simulink model "vehicle_spped_control_through_gear_input1"  (R2022a)
settings: Solver=VariableStepAuto  StartTime=0.0  StopTime=inf  RelTol=1e-3
settings Model: Creator=Admin  LastModifiedBy=Sanjana_Bagewadi
settings SolverCC: AlgebraicLoopSolver=TrustRegion
settings DebuggingCC: SFMachineParentedDataDiag=warning
settings RTWCC: DLArmComputeVersion=19.05

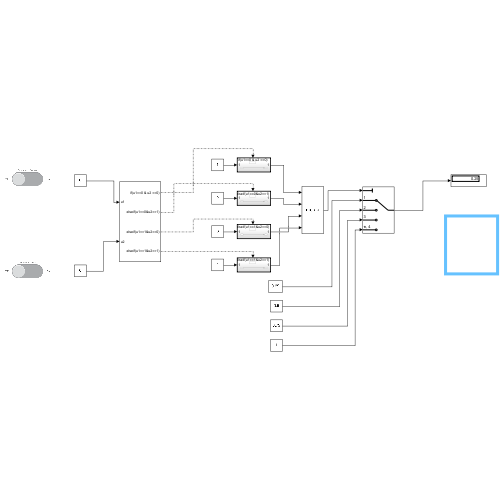
[thumbnail: Simulink's stored preview of the top-level diagram]
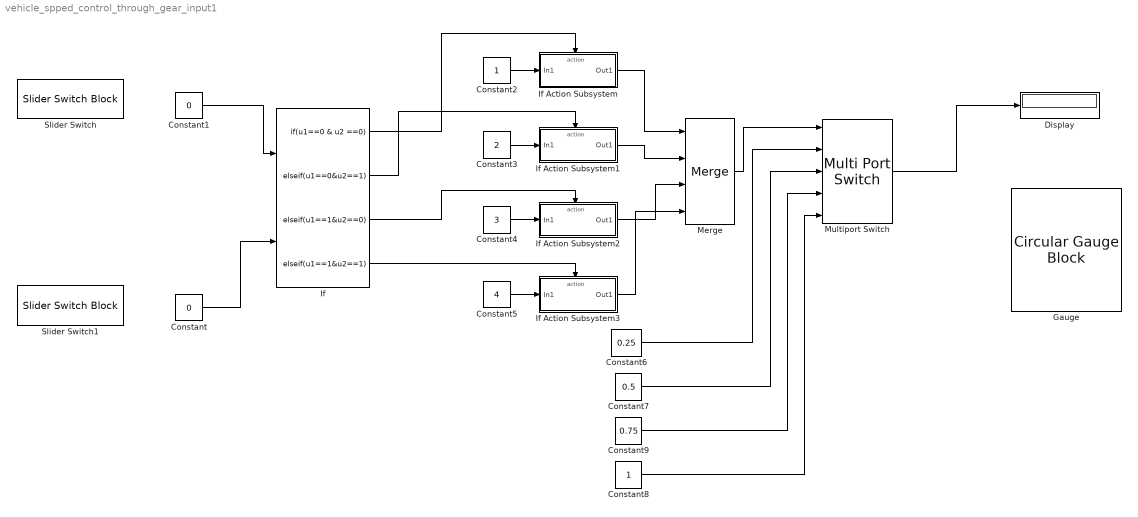
== system vehicle_spped_control_through_gear_input1 ==
  Constant : Constant  Value=0
  Constant1 : Constant  Value=0
  Constant2 : Constant
  Constant3 : Constant  Value=2
  Constant4 : Constant  Value=3
  Constant5 : Constant  Value=4
  Constant6 : Constant  Value=0.25
  Constant7 : Constant  Value=0.5
  Constant8 : Constant
  Constant9 : Constant  Value=0.75
  Display : Display
  Gauge : CircularGaugeBlock  ScaleMax=1
  If : If  NumInputs=2  IfExpression=u1==0 & u2 ==0  ElseIfExpressions=u1==0&u2==1,u1==1&u2==0,u1==1&u2==1  ShowElse=off
  If Action Subsystem : Subsystem  TreatAsAtomicUnit=on
  If Action Subsystem1 : Subsystem  TreatAsAtomicUnit=on
  If Action Subsystem2 : Subsystem  TreatAsAtomicUnit=on
  If Action Subsystem3 : Subsystem  TreatAsAtomicUnit=on
  Merge : Merge  Inputs=4
  Multiport Switch : MultiPortSwitch  Inputs=4  SaturateOnIntegerOverflow=off  InputSameDT=off
  Slider Switch : SliderSwitchBlock
      settings: Values={{'Off', 'On'}, [0 1]}
  Slider Switch1 : SliderSwitchBlock
      settings: Values={{'Off', 'On'}, [0 1]}
  wires:
  Constant1/1 -> If/1
  Constant/1 -> If/2
  If/1 -> If Action Subsystem/Action
  If/2 -> If Action Subsystem1/Action
  If/3 -> If Action Subsystem2/Action
  If/4 -> If Action Subsystem3/Action
  Constant2/1 -> If Action Subsystem/1(In1)
  Constant3/1 -> If Action Subsystem1/1(In1)
  Constant4/1 -> If Action Subsystem2/1(In1)
  Constant5/1 -> If Action Subsystem3/1(In1)
  If Action Subsystem/1(Out1) -> Merge/1
  If Action Subsystem1/1(Out1) -> Merge/2
  If Action Subsystem2/1(Out1) -> Merge/3
  If Action Subsystem3/1(Out1) -> Merge/4
  Constant7/1 -> Multiport Switch/3
  Multiport Switch/1 -> Display/1
  Constant8/1 -> Multiport Switch/5
  Constant6/1 -> Multiport Switch/2
  Constant9/1 -> Multiport Switch/4
  Merge/1 -> Multiport Switch/1

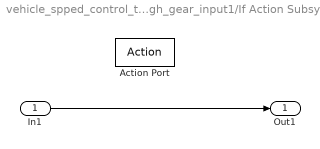
== system vehicle_spped_control_through_gear_input1/If Action Subsystem ==
  In1 : Inport
  Action Port : ActionPort  ActionPortLabel=if(u1==0 & u2 ==0)
  Out1 : Outport
  wires:
  In1/1 -> Out1/1

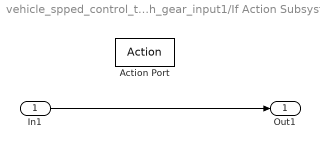
== system vehicle_spped_control_through_gear_input1/If Action Subsystem1 ==
  In1 : Inport
  Action Port : ActionPort  ActionPortLabel=elseif(u1==0&u2==1)
  Out1 : Outport
  wires:
  In1/1 -> Out1/1

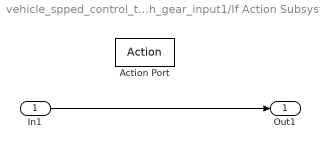
== system vehicle_spped_control_through_gear_input1/If Action Subsystem2 ==
  In1 : Inport
  Action Port : ActionPort  ActionPortLabel=elseif(u1==1&u2==0)
  Out1 : Outport
  wires:
  In1/1 -> Out1/1

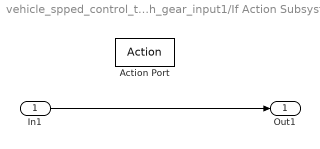
== system vehicle_spped_control_through_gear_input1/If Action Subsystem3 ==
  In1 : Inport
  Action Port : ActionPort  ActionPortLabel=elseif(u1==1&u2==1)
  Out1 : Outport
  wires:
  In1/1 -> Out1/1
